simulink model "REALTIME_PART2_robust_exact"  (R2020b)
settings: Solver=ode3  StartTime=0.0  StopTime=5  FixedStep=0.001  RelTol=1e-3
undefined symbols (not defined in the file or in its folder): ctrl, degs2rpm, denHws, denKi, GAMMA, H0, J0, Ke, Ki, N_u, N_x, National_Instruments, numHws, numKi, PCI, PHI, sens, step_size, T
libraries: sldrtlib x2
settings Model: ExtModeTrigDuration=6000  Creator=utente  LastModifiedBy=pavarinlau
settings DataIOCC: ReturnWorkspaceOutputs=off
settings RTWCC: Description=Simulink Desktop Real-Time  SystemTargetFile=sldrt.tlc  TemplateMakefile=sldrt.tmf  RTWCompilerOptimization=on
settings CodeAppCC: MaxIdLength=95
settings SimulinkDesktopRealTimeCC: TargetPreCompLibLocation=C:\Program Files\MATLAB\R2020b\toolbox\sldrt\lib\win64

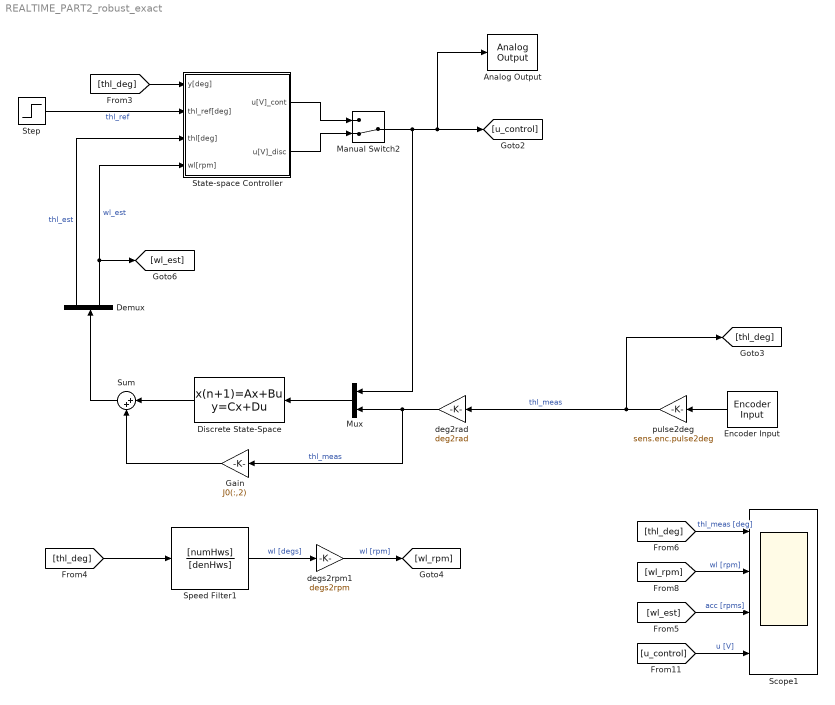
== system REALTIME_PART2_robust_exact ==
  Analog Output : sldrtlib/Analog Output  SampleTime=-1  MaxMissedTicks=10  ShowMissedTicks=off  YieldWhenWaiting=off  DrvName=National_Instruments/PCI-6221  DrvAddress=4294967295  DrvOptions=[0 0 0 2 0]  Channels=1  RangeMode=1  VoltRange=1  InitialValue=0  FinalValue=0
      settings: AttributesFormatString=National Instruments\nPCI-6221 [auto]
  Demux : Demux  Outputs=2
  Discrete State-Space : DiscreteStateSpace  A=PHI  B=GAMMA  C=H0  D=[0 0; 0 0]  SampleTime=T
  Encoder Input : sldrtlib/Encoder Input  SampleTime=T  MaxMissedTicks=10  ShowMissedTicks=off  YieldWhenWaiting=off  DrvName=National_Instruments/PCI-6221  DrvAddress=4294967295  DrvOptions=[0 0 0 2 0]  Channels=1  QuadMode=3  IndexPulse=1  InputFilter=Inf  DataType=1
      settings: AttributesFormatString=National Instruments\nPCI-6221 [auto]
  Gain : Gain  Gain=J0(:,2)
  Manual Switch2 : ManualSwitch  CurrentSetting=0
  Mux : Mux  Inputs=2
  Scope1 : Scope  NumInputPorts=4
  Speed Filter1 : TransferFcn  Numerator=[numHws]  Denominator=[denHws]
  State-space Controller : Subsystem
  Step : Step  After=step_size  SampleTime=T
  Sum : Sum  Inputs=|++
  deg2rad : Gain  Gain=deg2rad
  degs2rpm1 : Gain  Gain=degs2rpm
  pulse2deg : Gain  Gain=sens.enc.pulse2deg
  wires:
  Step/1 -> State-space Controller/2(thl_ref[deg])  "thl_ref"
  pulse2deg/1 -> [thl_deg], deg2rad/1  "thl_meas"
  Mux/1 -> Discrete State-Space/1
  Demux/1 -> State-space Controller/3(thl[deg])  "thl_est"
  deg2rad/1 -> Gain/1, Mux/2  "thl_meas"
  Demux/2 -> State-space Controller/4(wl[rpm]), [wl_est]  "wl_est"
  [thl_deg] -> State-space Controller/1(y[deg])
  State-space Controller/1(u[V]_cont) -> Manual Switch2/1
  State-space Controller/2(u[V]_disc) -> Manual Switch2/2
  Manual Switch2/1 -> Analog Output/1, [u_control], Mux/1
  Encoder Input/1 -> pulse2deg/1
  [thl_deg] -> Scope1/1  "thl_meas [deg]"
  [wl_rpm] -> Scope1/2  "wl [rpm]"
  [wl_est] -> Scope1/3  "acc [rpms]"
  [u_control] -> Scope1/4  "u [V]"
  Speed Filter1/1 -> degs2rpm1/1  "wl [degs]"
  [thl_deg] -> Speed Filter1/1
  degs2rpm1/1 -> [wl_rpm]  "wl [rpm]"
  Discrete State-Space/1 -> Sum/1
  Sum/1 -> Demux/1
  Gain/1 -> Sum/2

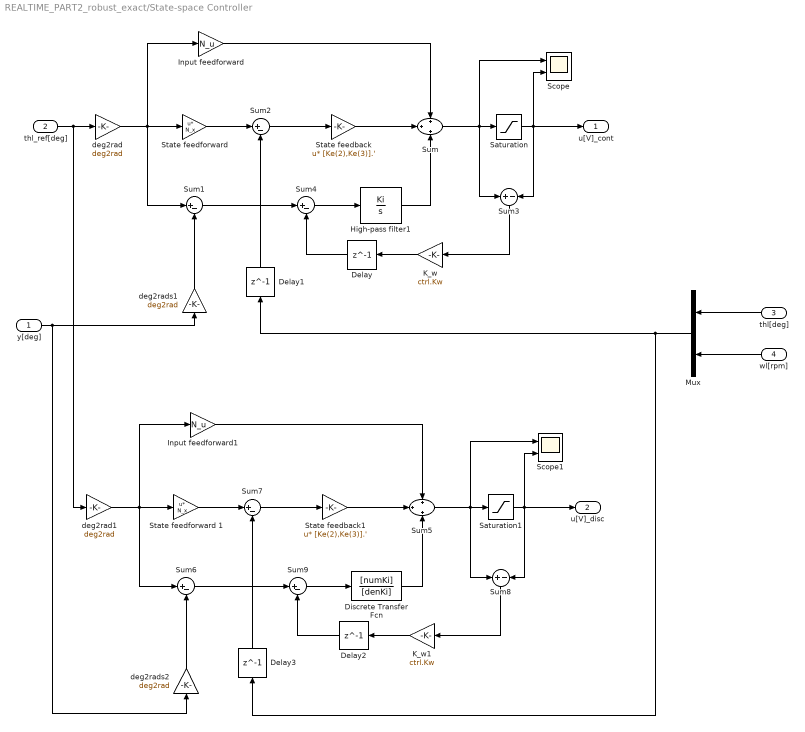
== system REALTIME_PART2_robust_exact/State-space Controller ==
  y[deg] : Inport
  thl_ref[deg] : Inport  Port=2
  thl[deg] : Inport  Port=3
  wl[rpm] : Inport  Port=4
  Delay{,1..3} (4 alike) : Delay  DelayLength=1  InitialCondition=0
  Discrete Transfer Fcn : DiscreteTransferFcn  Numerator=[numKi]  Denominator=[denKi]  SampleTime=T
  High-pass filter1 : TransferFcn  Numerator=Ki  Denominator=[1 0]
  Input feedforward : Gain  Gain=N_u
  Input feedforward1 : Gain  Gain=N_u
  K_w : Gain  Gain=ctrl.Kw
  K_w1 : Gain  Gain=ctrl.Kw
  Mux : Mux  Inputs=2
  Saturation : Saturate  UpperLimit=10  LowerLimit=-10
  Saturation1 : Saturate  UpperLimit=10  LowerLimit=-10
  Scope : Scope  NumInputPorts=2
  Scope1 : Scope  NumInputPorts=2
  State feedback : Gain  Gain=[Ke(2),Ke(3)].'  Multiplication=Matrix(u*K)
  State feedback1 : Gain  Gain=[Ke(2),Ke(3)].'  Multiplication=Matrix(u*K)
  "State feedforward\t" : Gain  Gain=N_x  Multiplication=Matrix(u*K)
  State feedforward	1 : Gain  Gain=N_x  Multiplication=Matrix(u*K)
  Sum : Sum  Inputs=+|+|+
  Sum{1..2,4,6..7,9} (6 alike) : Sum  Inputs=|+-
  Sum3 : Sum  Inputs=+|-
  Sum5 : Sum  Inputs=+|+|+
  Sum8 : Sum  Inputs=+|-
  deg2rad : Gain  Gain=deg2rad
  deg2rad1 : Gain  Gain=deg2rad
  deg2rads1 : Gain  Gain=deg2rad
  deg2rads2 : Gain  Gain=deg2rad
  u[V]_cont : Outport
  u[V]_disc : Outport  Port=2
  wires:
  deg2rad/1 -> Sum1/1, Input feedforward/1, "State feedforward\t"/1
  State feedback/1 -> Sum/2
  "State feedforward\t"/1 -> Sum2/1
  Sum2/1 -> State feedback/1
  Input feedforward/1 -> Sum/1
  thl[deg]/1 -> Mux/1
  wl[rpm]/1 -> Mux/2
  Mux/1 -> Delay1/1, Delay3/1
  High-pass filter1/1 -> Sum/3
  Sum1/1 -> Sum4/1
  deg2rads1/1 -> Sum1/2
  Saturation/1 -> Sum3/2, Scope/2, u[V]_cont/1
  Sum3/1 -> K_w/1
  Sum/1 -> Sum3/1, Scope/1, Saturation/1
  Sum4/1 -> High-pass filter1/1
  K_w/1 -> Delay/1
  Delay/1 -> Sum4/2
  Delay1/1 -> Sum2/2
  Sum8/1 -> K_w1/1
  Sum9/1 -> Discrete Transfer Fcn/1
  y[deg]/1 -> deg2rads1/1, deg2rads2/1
  deg2rads2/1 -> Sum6/2
  K_w1/1 -> Delay2/1
  Sum5/1 -> Sum8/1, Scope1/1, Saturation1/1
  Sum6/1 -> Sum9/1
  Saturation1/1 -> Sum8/2, Scope1/2, u[V]_disc/1
  Input feedforward1/1 -> Sum5/1
  Delay2/1 -> Sum9/2
  State feedforward	1/1 -> Sum7/1
  State feedback1/1 -> Sum5/2
  Sum7/1 -> State feedback1/1
  deg2rad1/1 -> Sum6/1, Input feedforward1/1, State feedforward	1/1
  thl_ref[deg]/1 -> deg2rad1/1, deg2rad/1
  Delay3/1 -> Sum7/2
  Discrete Transfer Fcn/1 -> Sum5/3
